simulink library "Springs_Linear"  (R2020b)
settings: Solver=VariableStepAuto  StartTime=0.0  StopTime=10.0  RelTol=1e-3
undefined symbols (not defined in the file): Spring
libraries: fl_lib x6, Spring_Basics x6
Description:
  | Component of Simscape Vehicle Templates Library
  | 
  | Copyright 2018-2020 The MathWorks, Inc.
settings Model: Creator=smiller  LastModifiedBy=smiller
settings DataIOCC: ReturnWorkspaceOutputs=off
settings DebuggingCC: ArithmeticOperatorsInVariantConditions=warning
settings SFSimCC: CustomCodeUndefinedFunction=UseInterfaceOnly

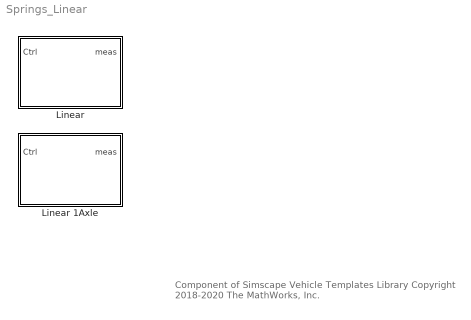
== system Springs_Linear ==
  note: Component of Simscape Vehicle Templates Library
      | Copyright 2018-2020 The MathWorks, Inc.
  Linear : Subsystem  VariantControl=Linear
  Linear 1Axle : Subsystem  VariantControl=Linear

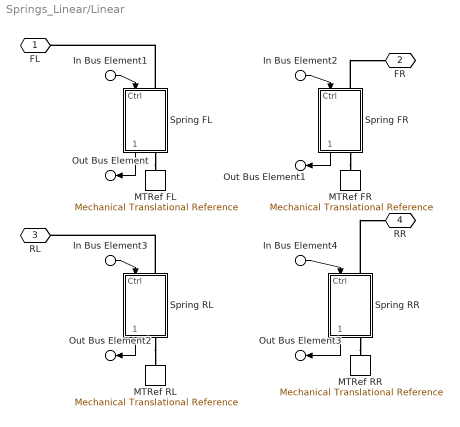
== system Springs_Linear/Linear ==
  In Bus Element1 : Inport  PortName=Ctrl  Element=FL
  In Bus Element2 : Inport  PortName=Ctrl  Element=FR
  In Bus Element3 : Inport  PortName=Ctrl  Element=RL
  In Bus Element4 : Inport  PortName=Ctrl  Element=RR
  MTRef FL : fl_lib/Mechanical/Translational Elements/Mechanical Translational Reference
  MTRef FR : fl_lib/Mechanical/Translational Elements/Mechanical Translational Reference
  MTRef RL : fl_lib/Mechanical/Translational Elements/Mechanical Translational Reference
  MTRef RR : fl_lib/Mechanical/Translational Elements/Mechanical Translational Reference
  Spring FL : Subsystem  mask{Spring=Spring.Front}
      mask prompts: Spring "Spring Parameters"
  Spring FR : Subsystem  mask{Spring=Spring.Front}
      mask prompts: Spring "Spring Parameters"
  Spring RL : Subsystem  mask{Spring=Spring.Rear}
      mask prompts: Spring "Spring Parameters"
  Spring RR : Subsystem  mask{Spring=Spring.Rear}
      mask prompts: Spring "Spring Parameters"
  FL : PMIOPort  Side=Left
  FR : PMIOPort  Port=2  Side=Right
  RL : PMIOPort  Port=3  Side=Left
  RR : PMIOPort  Port=4  Side=Right
  Out Bus Element : Outport  VectorParamsAs1DForOutWhenUnconnected=off  PortName=meas  Element=FL
  Out Bus Element1 : Outport  VectorParamsAs1DForOutWhenUnconnected=off  PortName=meas  Element=FR
  Out Bus Element2 : Outport  VectorParamsAs1DForOutWhenUnconnected=off  PortName=meas  Element=RL
  Out Bus Element3 : Outport  VectorParamsAs1DForOutWhenUnconnected=off  PortName=meas  Element=RR
  wires:
  In Bus Element1/1 -> Spring FL/1(Ctrl)
  Spring FL/1(Out1) -> Out Bus Element/1
  In Bus Element2/1 -> Spring FR/1(Ctrl)
  Spring FR/1(Out1) -> Out Bus Element1/1
  In Bus Element3/1 -> Spring RL/1(Ctrl)
  Spring RL/1(Out1) -> Out Bus Element2/1
  In Bus Element4/1 -> Spring RR/1(Ctrl)
  Spring RR/1(Out1) -> Out Bus Element3/1
  connections:
  Spring FR/LConn1 -- FR/RConn1
  Spring FR/RConn1 -- MTRef FR/LConn1
  Spring RR/LConn1 -- RR/RConn1
  Spring RR/RConn1 -- MTRef RR/LConn1
  Spring RL/LConn1 -- RL/RConn1
  Spring RL/RConn1 -- MTRef RL/LConn1
  Spring FL/LConn1 -- FL/RConn1
  Spring FL/RConn1 -- MTRef FL/LConn1

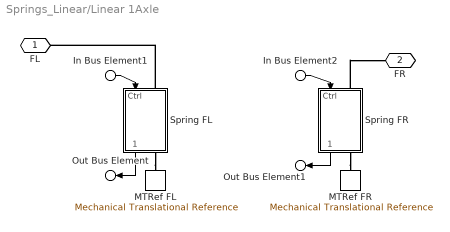
== system Springs_Linear/Linear 1Axle ==
  In Bus Element1 : Inport  PortName=Ctrl  Element=FL
  In Bus Element2 : Inport  PortName=Ctrl  Element=FR
  MTRef FL : fl_lib/Mechanical/Translational Elements/Mechanical Translational Reference
  MTRef FR : fl_lib/Mechanical/Translational Elements/Mechanical Translational Reference
  Spring FL : Subsystem  mask{Spring=Spring.Front}
      mask prompts: Spring "Spring Parameters"
  Spring FR : Subsystem  mask{Spring=Spring.Front}
      mask prompts: Spring "Spring Parameters"
  FL : PMIOPort  Side=Left
  FR : PMIOPort  Port=2  Side=Right
  Out Bus Element : Outport  VectorParamsAs1DForOutWhenUnconnected=off  PortName=meas  Element=FL
  Out Bus Element1 : Outport  VectorParamsAs1DForOutWhenUnconnected=off  PortName=meas  Element=FR
  wires:
  Spring FR/1(Out1) -> Out Bus Element1/1
  In Bus Element2/1 -> Spring FR/1(Ctrl)
  Spring FL/1(Out1) -> Out Bus Element/1
  In Bus Element1/1 -> Spring FL/1(Ctrl)
  connections:
  Spring FL/RConn1 -- MTRef FL/LConn1
  Spring FL/LConn1 -- FL/RConn1
  Spring FR/RConn1 -- MTRef FR/LConn1
  Spring FR/LConn1 -- FR/RConn1

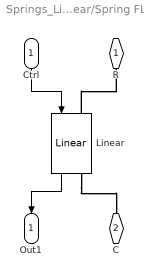
== system Springs_Linear/Linear/Spring FL ==
  Ctrl : Inport
  Linear : Spring_Basics/Linear  VariantControl=Linear  spr_def0=Spring.xPreload.Value  spr_k=Spring.K.Value  spr_hp_top=Spring.sTop.Value  spr_hp_bot=Spring.sBottom.Value
  R : PMIOPort  Side=Left
  C : PMIOPort  Port=2  Side=Right
  Out1 : Outport  VectorParamsAs1DForOutWhenUnconnected=off
  wires:
  Linear/1 -> Out1/1
  Ctrl/1 -> Linear/1
  connections:
  Linear/LConn1 -- R/RConn1
  Linear/RConn1 -- C/RConn1

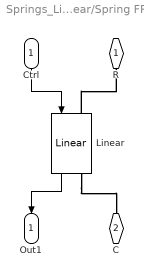
== system Springs_Linear/Linear/Spring FR ==
  Ctrl : Inport
  Linear : Spring_Basics/Linear  VariantControl=Linear  spr_def0=Spring.xPreload.Value  spr_k=Spring.K.Value  spr_hp_top=Spring.sTop.Value  spr_hp_bot=Spring.sBottom.Value
  R : PMIOPort  Side=Left
  C : PMIOPort  Port=2  Side=Right
  Out1 : Outport  VectorParamsAs1DForOutWhenUnconnected=off
  wires:
  Ctrl/1 -> Linear/1
  Linear/1 -> Out1/1
  connections:
  Linear/RConn1 -- C/RConn1
  Linear/LConn1 -- R/RConn1

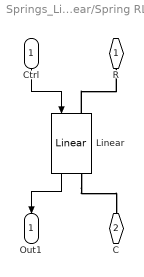
== system Springs_Linear/Linear/Spring RL ==
  Ctrl : Inport
  Linear : Spring_Basics/Linear  VariantControl=Linear  spr_def0=Spring.xPreload.Value  spr_k=Spring.K.Value  spr_hp_top=Spring.sTop.Value  spr_hp_bot=Spring.sBottom.Value
  R : PMIOPort  Side=Left
  C : PMIOPort  Port=2  Side=Right
  Out1 : Outport  VectorParamsAs1DForOutWhenUnconnected=off
  wires:
  Ctrl/1 -> Linear/1
  Linear/1 -> Out1/1
  connections:
  Linear/RConn1 -- C/RConn1
  Linear/LConn1 -- R/RConn1

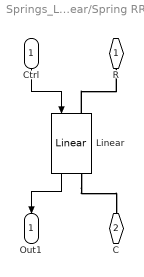
== system Springs_Linear/Linear/Spring RR ==
  Ctrl : Inport
  Linear : Spring_Basics/Linear  VariantControl=Linear  spr_def0=Spring.xPreload.Value  spr_k=Spring.K.Value  spr_hp_top=Spring.sTop.Value  spr_hp_bot=Spring.sBottom.Value
  R : PMIOPort  Side=Left
  C : PMIOPort  Port=2  Side=Right
  Out1 : Outport  VectorParamsAs1DForOutWhenUnconnected=off
  wires:
  Linear/1 -> Out1/1
  Ctrl/1 -> Linear/1
  connections:
  Linear/LConn1 -- R/RConn1
  Linear/RConn1 -- C/RConn1

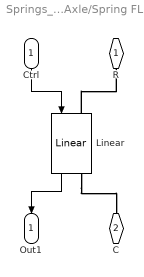
== system Springs_Linear/Linear 1Axle/Spring FL ==
  Ctrl : Inport
  Linear : Spring_Basics/Linear  VariantControl=Linear  spr_def0=Spring.xPreload.Value  spr_k=Spring.K.Value  spr_hp_top=Spring.sTop.Value  spr_hp_bot=Spring.sBottom.Value
  R : PMIOPort  Side=Left
  C : PMIOPort  Port=2  Side=Right
  Out1 : Outport  VectorParamsAs1DForOutWhenUnconnected=off
  wires:
  Ctrl/1 -> Linear/1
  Linear/1 -> Out1/1
  connections:
  Linear/RConn1 -- C/RConn1
  Linear/LConn1 -- R/RConn1

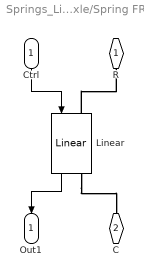
== system Springs_Linear/Linear 1Axle/Spring FR ==
  Ctrl : Inport
  Linear : Spring_Basics/Linear  VariantControl=Linear  spr_def0=Spring.xPreload.Value  spr_k=Spring.K.Value  spr_hp_top=Spring.sTop.Value  spr_hp_bot=Spring.sBottom.Value
  R : PMIOPort  Side=Left
  C : PMIOPort  Port=2  Side=Right
  Out1 : Outport  VectorParamsAs1DForOutWhenUnconnected=off
  wires:
  Linear/1 -> Out1/1
  Ctrl/1 -> Linear/1
  connections:
  Linear/LConn1 -- R/RConn1
  Linear/RConn1 -- C/RConn1
